simulink model "PID_MODEL"  (R2023b)
settings: Solver=FixedStepDiscrete  StartTime=0.0  StopTime=50  FixedStep=0.001  RelTol=1e-3
values from neighbouring files (symbols this model uses):
  ANG_A_D_CH1_1 = 0    [ini.m]
  ANG_A_D_CH1_2 = 0    [ini.m]
  ANG_A_D_CH1_3 = 0    [ini.m]
  ANG_A_D_CH1_4 = 0    [ini.m]
  ANG_A_D_CH1_5 = 0    [ini.m]
  ANG_A_D_CH1_6 = 0    [ini.m]
  ANG_A_D_CH1_7 = 0    [ini.m]
  ANG_A_D_CH2_1 = 0    [ini.m]
  ANG_A_D_CH2_2 = 0    [ini.m]
  ANG_A_D_CH2_3 = 0    [ini.m]
  ANG_A_D_CH2_4 = 0    [ini.m]
  ANG_A_D_CH2_5 = 0    [ini.m]
  ANG_A_D_CH2_6 = 0    [ini.m]
  ANG_A_D_CH2_7 = 0    [ini.m]
  ANG_A_I_CH1_1 = 0    [ini.m]
  ANG_A_I_CH1_2 = 0    [ini.m]
  ANG_A_I_CH1_3 = 0    [ini.m]
  ANG_A_I_CH1_4 = 0    [ini.m]
  ANG_A_I_CH1_5 = 0    [ini.m]
  ANG_A_I_CH1_6 = 0    [ini.m]
  ANG_A_I_CH1_7 = 0    [ini.m]
  ANG_A_I_CH2_1 = 0    [ini.m]
  ANG_A_I_CH2_2 = 0    [ini.m]
  ANG_A_I_CH2_3 = 0    [ini.m]
  ANG_A_I_CH2_4 = 0    [ini.m]
  ANG_A_I_CH2_5 = 0    [ini.m]
  ANG_A_I_CH2_6 = 0    [ini.m]
  ANG_A_I_CH2_7 = 0    [ini.m]
  ANG_A_P_CH1_1 = 0    [ini.m]
  ANG_A_P_CH1_2 = 0    [ini.m]
  ANG_A_P_CH1_3 = 0    [ini.m]
  ANG_A_P_CH1_4 = 0    [ini.m]
  ANG_A_P_CH1_5 = 0    [ini.m]
  ANG_A_P_CH1_6 = 0    [ini.m]
  ANG_A_P_CH1_7 = 0    [ini.m]
  ANG_A_P_CH2_1 = 0    [ini.m]
  ANG_A_P_CH2_2 = 0    [ini.m]
  ANG_A_P_CH2_3 = 0    [ini.m]
  ANG_A_P_CH2_4 = 0    [ini.m]
  ANG_A_P_CH2_5 = 0    [ini.m]
  ANG_A_P_CH2_6 = 0    [ini.m]
  ANG_A_P_CH2_7 = 0    [ini.m]
  ANG_S_D_CH1_1 = 0    [ini.m]
  ANG_S_D_CH1_2 = 0    [ini.m]
  ANG_S_D_CH1_3 = 0    [ini.m]
  ANG_S_D_CH1_4 = 0    [ini.m]
  ANG_S_D_CH1_5 = 0    [ini.m]
  ANG_S_D_CH1_6 = 0    [ini.m]
  ANG_S_D_CH1_7 = 0    [ini.m]
  ANG_S_D_CH2_1 = 0    [ini.m]
  ANG_S_D_CH2_2 = 0    [ini.m]
  ANG_S_D_CH2_3 = 0    [ini.m]
  ANG_S_D_CH2_4 = 0    [ini.m]
  ANG_S_D_CH2_5 = 0    [ini.m]
  ANG_S_D_CH2_6 = 0    [ini.m]
  ANG_S_D_CH2_7 = 0    [ini.m]
  ANG_S_I_CH1_1 = 0    [ini.m]
  ANG_S_I_CH1_2 = 0    [ini.m]
  ANG_S_I_CH1_3 = 0    [ini.m]
  ANG_S_I_CH1_4 = 0    [ini.m]
  ANG_S_I_CH1_5 = 0    [ini.m]
  ANG_S_I_CH1_6 = 0    [ini.m]
  ANG_S_I_CH1_7 = 0    [ini.m]
  ANG_S_I_CH2_1 = 0    [ini.m]
  ANG_S_I_CH2_2 = 0    [ini.m]
  ANG_S_I_CH2_3 = 0    [ini.m]
  ANG_S_I_CH2_4 = 0    [ini.m]
  ANG_S_I_CH2_5 = 0    [ini.m]
  ANG_S_I_CH2_6 = 0    [ini.m]
  ANG_S_I_CH2_7 = 0    [ini.m]
  ANG_S_P_CH1_1 = 0    [ini.m]
  ANG_S_P_CH1_2 = 0    [ini.m]
  ANG_S_P_CH1_3 = 0    [ini.m]
  ANG_S_P_CH1_4 = 0    [ini.m]
  ANG_S_P_CH1_5 = 0    [ini.m]
  ANG_S_P_CH1_6 = 0    [ini.m]
  ANG_S_P_CH1_7 = 0    [ini.m]
  ANG_S_P_CH2_1 = 0    [ini.m]
  ANG_S_P_CH2_2 = 0    [ini.m]
  ANG_S_P_CH2_3 = 0    [ini.m]
  ANG_S_P_CH2_4 = 0    [ini.m]
  ANG_S_P_CH2_5 = 0    [ini.m]
  ANG_S_P_CH2_6 = 0    [ini.m]
  ANG_S_P_CH2_7 = 0    [ini.m]
  DEADBAND_CH1_1 = 500    [ini.m]
  DEADBAND_CH1_2 = 500    [ini.m]
  DEADBAND_CH1_3 = 500    [ini.m]
  DEADBAND_CH1_4 = 500    [ini.m]
  DEADBAND_CH1_5 = 500    [ini.m]
  DEADBAND_CH1_6 = 500    [ini.m]
  DEADBAND_CH1_7 = 500    [ini.m]
  DEADBAND_CH2_1 = 500    [ini.m]
  DEADBAND_CH2_2 = 500    [ini.m]
  DEADBAND_CH2_3 = 500    [ini.m]
  DEADBAND_CH2_4 = 500    [ini.m]
  DEADBAND_CH2_5 = 500    [ini.m]
  DEADBAND_CH2_6 = 500    [ini.m]
  DEADBAND_CH2_7 = 500    [ini.m]
  SPD_D_CH1_1 = 0    [ini.m]
  SPD_D_CH1_2 = 0    [ini.m]
  SPD_D_CH1_3 = 0    [ini.m]
  SPD_D_CH1_4 = 0    [ini.m]
  SPD_D_CH1_5 = 0    [ini.m]
  SPD_D_CH1_6 = 0    [ini.m]
  SPD_D_CH1_7 = 0    [ini.m]
  SPD_D_CH2_1 = 0    [ini.m]
  SPD_D_CH2_2 = 0    [ini.m]
  SPD_D_CH2_3 = 0    [ini.m]
  SPD_D_CH2_4 = 0    [ini.m]
  SPD_D_CH2_5 = 0    [ini.m]
  SPD_D_CH2_6 = 0    [ini.m]
  SPD_D_CH2_7 = 0    [ini.m]
  SPD_I_CH1_1 = 0    [ini.m]
  SPD_I_CH1_2 = 0    [ini.m]
  SPD_I_CH1_3 = 0    [ini.m]
  SPD_I_CH1_4 = 0    [ini.m]
  SPD_I_CH1_5 = 0    [ini.m]
  SPD_I_CH1_6 = 0    [ini.m]
  SPD_I_CH1_7 = 0    [ini.m]
  SPD_I_CH2_1 = 0    [ini.m]
  ... (+34 more)
libraries: slpidlib x42
(part 5 of 5)

== system PID_MODEL/Yaw_CH2_5/If Action_speed Subsystem ==
  yaw_speed_rpm : Inport  OutDataTypeStr=single
  yaw_target : Inport  Port=2  OutDataTypeStr=single
  Action Port : ActionPort  ActionPortLabel=case [ 1 ]:
  Discrete PID Controller1 : slpidlib/PID Controller  Controller=PID  Form=Parallel  TimeDomain=Discrete-time  UseExternalTs=off  SampleTime=-1  IntegratorMethod=Forward Euler  FilterMethod=Forward Euler  ControllerParametersSource=internal  P=SPD_P_CH2_5  I=SPD_I_CH2_5  UseKiTs=off  D=SPD_D_CH2_5  N=100  UseFilter=on  TunerSelectOption=Transfer Function Based (PID Tuner App)  InitialConditionSource=internal  InitialConditionForIntegrator=0  InitialConditionForFilter=0  DifferentiatorICPrevScaledInput=0  ExternalReset=none  TrackingMode=off  Kt=1  LimitOutput=on  SatLimitsSource=internal  UpperSaturationLimit=16384  LowerSaturationLimit=-16384  LinearizeAsGain=off  AntiWindupMode=none  Kb=1  LimitIntegrator=off  UpperIntegratorSaturationLimit=inf  LowerIntegratorSaturationLimit=-inf  POutMin=[]  POutMax=[]  IOutMin=[]  IOutMax=[]  DOutMin=[]  DOutMax=[]  NOutMin=[]  NOutMax=[]  SumOutMin=[]  SumOutMax=[]  SaturationOutMin=[]  SaturationOutMax=[]  PParamMin=[]  PParamMax=[]  IParamMin=[]  IParamMax=[]  DParamMin=[]  DParamMax=[]  NParamMin=[]  NParamMax=[]  KbParamMin=[]  KbParamMax=[]  KtParamMin=[]  KtParamMax=[]  KbOutMin=[]  KbOutMax=[]  KtOutMin=[]  KtOutMax=[]  IntegratorOutMin=[]  IntegratorOutMax=[]  FilterOutMin=[]  FilterOutMax=[]  SumI1OutMin=[]  SumI1OutMax=[]  SumI2OutMin=[]  SumI2OutMax=[]  SumI3OutMin=[]  SumI3OutMax=[]  SumI4OutMin=[]  SumI4OutMax=[]  SumDOutMin=[]  SumDOutMax=[]  DifferentiatorOutMin=[]  DifferentiatorOutMax=[]  FilterDiffOutCoefMin=[]  FilterDiffOutCoefMax=[]  ReciprocalOutMin=[]  ReciprocalOutMax=[]  SumDenOutMin=[]  SumDenOutMax=[]  SumNumOutMin=[]  SumNumOutMax=[]  DivideOutMin=[]  DivideOutMax=[]  UdiffTsProdOutMin=[]  UdiffTsProdOutMax=[]  NTsProdOutMin=[]  NTsProdOutMax=[]  UintegralTsProdOutMin=[]  UintegralTsProdOutMax=[]  UngainTsProdOutMin=[]  UngainTsProdOutMax=[]  ClampingZeroOutDataTypeStr=Inherit: Inherit via back propagation  ClampingZeroOutMin=[]  ClampingZeroOutMax=[]  FilterDenConstantOutDataTypeStr=Inherit: Inherit via back propagation  FilterDenConstantOutMin=[]  FilterDenConstantOutMax=[]  PCopyOutDataTypeStr=Inherit: Inherit via back propagation  PCopyOutMin=[]  PCopyOutMax=[]  NCopyOutDataTypeStr=Inherit: Inherit via back propagation  NCopyOutMin=[]  NCopyOutMax=[]  IntegratorContinuousStateAttributes=''  IntegratorStateMustResolveToSignalObject=off  IntegratorRTWStateStorageClass=Auto  FilterContinuousStateAttributes=''  FilterStateMustResolveToSignalObject=off  FilterRTWStateStorageClass=Auto  ParallelPVariant=InternalParameters  IdealPVariant=Disabled  IVariant=InternalParameters  DVariant=InternalParameters  IntegratorVariant=Discrete  SatVariant=Enabled  AWVariant=Passthrough  PCopyVariant=Disabled  TRVariant=Disabled  FdbkBlocksVariant=Forward  IdealPFdbkVariant=Disabled  SatFdbkVariant=Disabled  DerivativeFilterVariant=ForwardEulerFilter  NVariant=InternalParameters  NCopyVariant=Disabled  FilterICVariant=InternalICsFilter  IntegratorICVariant=InternalICs  ExternalResetVariant=Disabled  TRSumVariant=Passthrough  SumFdbkVariant=Disabled  SumVariant=Sum_PID  TsampFilterVariant=InternalTs  TsampNgainVariant=Passthrough  TsampIntegralVariant=Disabled_SignalSpec  ExternalSaturationOutDataTypeStr=Inherit: Same as second input
      settings: LibrarySourceBlock=simulink/Discrete/Discrete PID Controller
  Sum : Sum  Inputs=|+-  OutDataTypeStr=single
  Out1 : Outport  OutDataTypeStr=single
  wires:
  yaw_speed_rpm/1 -> Sum/2
  yaw_target/1 -> Sum/1
  Sum/1 -> Discrete PID Controller1/1
  Discrete PID Controller1/1 -> Out1/1

== system PID_MODEL/Yaw_CH2_5/If Action_speed Subsystem1 ==
  yaw_speed_rpm : Inport  OutDataTypeStr=single
  yaw_target : Inport  Port=2  OutDataTypeStr=single
  yaw_ecd : Inport  Port=3  OutDataTypeStr=single
  yaw_last_ecd : Inport  Port=4  OutDataTypeStr=single
  yaw_circle : Inport  Port=5  OutDataTypeStr=single
  Action Port : ActionPort  ActionPortLabel=case [ 2 ]:
  Abs : Abs  OutDataTypeStr=single  SaturateOnIntegerOverflow=off
  Chart1 : Stateflow chart  TreatAsAtomicUnit=on
  Constant : Constant  Value=0  OutDataTypeStr=single
  Discrete PID Controller : slpidlib/PID Controller  Controller=PID  Form=Parallel  TimeDomain=Discrete-time  UseExternalTs=off  SampleTime=-1  IntegratorMethod=Forward Euler  FilterMethod=Forward Euler  ControllerParametersSource=internal  P=ANG_S_P_CH2_5  I=ANG_S_I_CH2_5  UseKiTs=off  D=ANG_S_D_CH2_5  N=100  UseFilter=on  TunerSelectOption=Transfer Function Based (PID Tuner App)  InitialConditionSource=internal  InitialConditionForIntegrator=0  InitialConditionForFilter=0  DifferentiatorICPrevScaledInput=0  ExternalReset=none  TrackingMode=off  Kt=1  LimitOutput=on  SatLimitsSource=internal  UpperSaturationLimit=16384  LowerSaturationLimit=-16384  LinearizeAsGain=off  AntiWindupMode=none  Kb=1  LimitIntegrator=off  UpperIntegratorSaturationLimit=2000  LowerIntegratorSaturationLimit=-2000  POutMin=[]  POutMax=[]  IOutMin=[]  IOutMax=[]  DOutMin=[]  DOutMax=[]  NOutMin=[]  NOutMax=[]  SumOutMin=[]  SumOutMax=[]  SaturationOutMin=[]  SaturationOutMax=[]  PParamMin=[]  PParamMax=[]  IParamMin=[]  IParamMax=[]  DParamMin=[]  DParamMax=[]  NParamMin=[]  NParamMax=[]  KbParamMin=[]  KbParamMax=[]  KtParamMin=[]  KtParamMax=[]  KbOutMin=[]  KbOutMax=[]  KtOutMin=[]  KtOutMax=[]  IntegratorOutMin=[]  IntegratorOutMax=[]  FilterOutMin=[]  FilterOutMax=[]  SumI1OutMin=[]  SumI1OutMax=[]  SumI2OutMin=[]  SumI2OutMax=[]  SumI3OutMin=[]  SumI3OutMax=[]  SumI4OutMin=[]  SumI4OutMax=[]  SumDOutMin=[]  SumDOutMax=[]  DifferentiatorOutMin=[]  DifferentiatorOutMax=[]  FilterDiffOutCoefMin=[]  FilterDiffOutCoefMax=[]  ReciprocalOutMin=[]  ReciprocalOutMax=[]  SumDenOutMin=[]  SumDenOutMax=[]  SumNumOutMin=[]  SumNumOutMax=[]  DivideOutMin=[]  DivideOutMax=[]  UdiffTsProdOutMin=[]  UdiffTsProdOutMax=[]  NTsProdOutMin=[]  NTsProdOutMax=[]  UintegralTsProdOutMin=[]  UintegralTsProdOutMax=[]  UngainTsProdOutMin=[]  UngainTsProdOutMax=[]  ClampingZeroOutDataTypeStr=Inherit: Inherit via back propagation  ClampingZeroOutMin=[]  ClampingZeroOutMax=[]  FilterDenConstantOutDataTypeStr=Inherit: Inherit via back propagation  FilterDenConstantOutMin=[]  FilterDenConstantOutMax=[]  PCopyOutDataTypeStr=Inherit: Inherit via back propagation  PCopyOutMin=[]  PCopyOutMax=[]  NCopyOutDataTypeStr=Inherit: Inherit via back propagation  NCopyOutMin=[]  NCopyOutMax=[]  IntegratorContinuousStateAttributes=''  IntegratorStateMustResolveToSignalObject=off  IntegratorRTWStateStorageClass=Auto  FilterContinuousStateAttributes=''  FilterStateMustResolveToSignalObject=off  FilterRTWStateStorageClass=Auto  ParallelPVariant=InternalParameters  IdealPVariant=Disabled  IVariant=InternalParameters  DVariant=InternalParameters  IntegratorVariant=Discrete  SatVariant=Enabled  AWVariant=Passthrough  PCopyVariant=Disabled  TRVariant=Disabled  FdbkBlocksVariant=Forward  IdealPFdbkVariant=Disabled  SatFdbkVariant=Disabled  DerivativeFilterVariant=ForwardEulerFilter  NVariant=InternalParameters  NCopyVariant=Disabled  FilterICVariant=InternalICsFilter  IntegratorICVariant=InternalICs  ExternalResetVariant=Disabled  TRSumVariant=Passthrough  SumFdbkVariant=Disabled  SumVariant=Sum_PID  TsampFilterVariant=InternalTs  TsampNgainVariant=Passthrough  TsampIntegralVariant=Disabled_SignalSpec  ExternalSaturationOutDataTypeStr=Inherit: Same as second input
      settings: LibrarySourceBlock=simulink/Discrete/Discrete PID Controller
  Discrete PID Controller1 : slpidlib/PID Controller  Controller=PID  Form=Parallel  TimeDomain=Discrete-time  UseExternalTs=off  SampleTime=-1  IntegratorMethod=Forward Euler  FilterMethod=Forward Euler  ControllerParametersSource=internal  P=ANG_A_P_CH2_5  I=ANG_A_I_CH2_5  UseKiTs=off  D=ANG_A_D_CH2_5  N=100  UseFilter=on  TunerSelectOption=Transfer Function Based (PID Tuner App)  InitialConditionSource=internal  InitialConditionForIntegrator=0  InitialConditionForFilter=0  DifferentiatorICPrevScaledInput=0  ExternalReset=none  TrackingMode=off  Kt=1  LimitOutput=on  SatLimitsSource=internal  UpperSaturationLimit=16384  LowerSaturationLimit=-16384  LinearizeAsGain=off  AntiWindupMode=none  Kb=1  LimitIntegrator=off  UpperIntegratorSaturationLimit=500  LowerIntegratorSaturationLimit=-500  POutMin=[]  POutMax=[]  IOutMin=[]  IOutMax=[]  DOutMin=[]  DOutMax=[]  NOutMin=[]  NOutMax=[]  SumOutMin=[]  SumOutMax=[]  SaturationOutMin=[]  SaturationOutMax=[]  PParamMin=[]  PParamMax=[]  IParamMin=[]  IParamMax=[]  DParamMin=[]  DParamMax=[]  NParamMin=[]  NParamMax=[]  KbParamMin=[]  KbParamMax=[]  KtParamMin=[]  KtParamMax=[]  KbOutMin=[]  KbOutMax=[]  KtOutMin=[]  KtOutMax=[]  IntegratorOutMin=[]  IntegratorOutMax=[]  FilterOutMin=[]  FilterOutMax=[]  SumI1OutMin=[]  SumI1OutMax=[]  SumI2OutMin=[]  SumI2OutMax=[]  SumI3OutMin=[]  SumI3OutMax=[]  SumI4OutMin=[]  SumI4OutMax=[]  SumDOutMin=[]  SumDOutMax=[]  DifferentiatorOutMin=[]  DifferentiatorOutMax=[]  FilterDiffOutCoefMin=[]  FilterDiffOutCoefMax=[]  ReciprocalOutMin=[]  ReciprocalOutMax=[]  SumDenOutMin=[]  SumDenOutMax=[]  SumNumOutMin=[]  SumNumOutMax=[]  DivideOutMin=[]  DivideOutMax=[]  UdiffTsProdOutMin=[]  UdiffTsProdOutMax=[]  NTsProdOutMin=[]  NTsProdOutMax=[]  UintegralTsProdOutMin=[]  UintegralTsProdOutMax=[]  UngainTsProdOutMin=[]  UngainTsProdOutMax=[]  ClampingZeroOutDataTypeStr=Inherit: Inherit via back propagation  ClampingZeroOutMin=[]  ClampingZeroOutMax=[]  FilterDenConstantOutDataTypeStr=Inherit: Inherit via back propagation  FilterDenConstantOutMin=[]  FilterDenConstantOutMax=[]  PCopyOutDataTypeStr=Inherit: Inherit via back propagation  PCopyOutMin=[]  PCopyOutMax=[]  NCopyOutDataTypeStr=Inherit: Inherit via back propagation  NCopyOutMin=[]  NCopyOutMax=[]  IntegratorContinuousStateAttributes=''  IntegratorStateMustResolveToSignalObject=off  IntegratorRTWStateStorageClass=Auto  FilterContinuousStateAttributes=''  FilterStateMustResolveToSignalObject=off  FilterRTWStateStorageClass=Auto  ParallelPVariant=InternalParameters  IdealPVariant=Disabled  IVariant=InternalParameters  DVariant=InternalParameters  IntegratorVariant=Discrete  SatVariant=Enabled  AWVariant=Passthrough  PCopyVariant=Disabled  TRVariant=Disabled  FdbkBlocksVariant=Forward  IdealPFdbkVariant=Disabled  SatFdbkVariant=Disabled  DerivativeFilterVariant=ForwardEulerFilter  NVariant=InternalParameters  NCopyVariant=Disabled  FilterICVariant=InternalICsFilter  IntegratorICVariant=InternalICs  ExternalResetVariant=Disabled  TRSumVariant=Passthrough  SumFdbkVariant=Disabled  SumVariant=Sum_PID  TsampFilterVariant=InternalTs  TsampNgainVariant=Passthrough  TsampIntegralVariant=Disabled_SignalSpec  ExternalSaturationOutDataTypeStr=Inherit: Same as second input
      settings: LibrarySourceBlock=simulink/Discrete/Discrete PID Controller
  Gain : Gain  Gain=8191  OutDataTypeStr=single
  Multiply : Gain  Gain=TRANS_CH2_5  OutDataTypeStr=single
  Sum : Sum  Inputs=|+-  OutDataTypeStr=single
  Sum1 : Sum  Inputs=|+-  OutDataTypeStr=single
  Sum2 : Sum  Inputs=|++  OutDataTypeStr=single
  Sum3 : Sum  Inputs=|+-  OutDataTypeStr=single
  Sum4 : Sum  Inputs=|++  OutDataTypeStr=single
  Switch1 : Switch  Criteria=u2 > Threshold  Threshold=DEADBAND_CH2_5  OutDataTypeStr=single  SaturateOnIntegerOverflow=off  InputSameDT=off
  Switch2 : Switch  Criteria=u2 > Threshold  Threshold=DEADBAND_CH2_5  OutDataTypeStr=single  SaturateOnIntegerOverflow=off  InputSameDT=off
  Out1 : Outport  OutDataTypeStr=single
  yaw_circle_out : Outport  Port=2  OutDataTypeStr=single
  wires:
  yaw_target/1 -> Sum/1
  Discrete PID Controller1/1 -> Multiply/1
  yaw_circle/1 -> Sum4/2, Gain/1
  Gain/1 -> Sum2/1
  yaw_ecd/1 -> Sum2/2, Sum3/1
  Sum2/1 -> Sum/2
  yaw_last_ecd/1 -> Sum3/2
  Sum3/1 -> Chart1/1(u1)
  Chart1/1(u2) -> Sum4/1
  Sum4/1 -> yaw_circle_out/1
  Multiply/1 -> Sum1/1
  Sum1/1 -> Switch1/1
  yaw_speed_rpm/1 -> Sum1/2
  Discrete PID Controller/1 -> Out1/1
  Switch1/1 -> Discrete PID Controller/1
  Abs/1 -> Switch2/2, Switch1/2
  Constant/1 -> Switch2/3, Switch1/3
  Sum/1 -> Switch2/1, Abs/1
  Switch2/1 -> Discrete PID Controller1/1

== system PID_MODEL/Yaw_CH2_6/If Action_speed Subsystem ==
  yaw_speed_rpm : Inport  OutDataTypeStr=single
  yaw_target : Inport  Port=2  OutDataTypeStr=single
  Action Port : ActionPort  ActionPortLabel=case [ 1 ]:
  Discrete PID Controller1 : slpidlib/PID Controller  Controller=PID  Form=Parallel  TimeDomain=Discrete-time  UseExternalTs=off  SampleTime=-1  IntegratorMethod=Forward Euler  FilterMethod=Forward Euler  ControllerParametersSource=internal  P=SPD_P_CH2_6  I=SPD_I_CH2_6  UseKiTs=off  D=SPD_D_CH2_6  N=100  UseFilter=on  TunerSelectOption=Transfer Function Based (PID Tuner App)  InitialConditionSource=internal  InitialConditionForIntegrator=0  InitialConditionForFilter=0  DifferentiatorICPrevScaledInput=0  ExternalReset=none  TrackingMode=off  Kt=1  LimitOutput=on  SatLimitsSource=internal  UpperSaturationLimit=16384  LowerSaturationLimit=-16384  LinearizeAsGain=off  AntiWindupMode=none  Kb=1  LimitIntegrator=off  UpperIntegratorSaturationLimit=inf  LowerIntegratorSaturationLimit=-inf  POutMin=[]  POutMax=[]  IOutMin=[]  IOutMax=[]  DOutMin=[]  DOutMax=[]  NOutMin=[]  NOutMax=[]  SumOutMin=[]  SumOutMax=[]  SaturationOutMin=[]  SaturationOutMax=[]  PParamMin=[]  PParamMax=[]  IParamMin=[]  IParamMax=[]  DParamMin=[]  DParamMax=[]  NParamMin=[]  NParamMax=[]  KbParamMin=[]  KbParamMax=[]  KtParamMin=[]  KtParamMax=[]  KbOutMin=[]  KbOutMax=[]  KtOutMin=[]  KtOutMax=[]  IntegratorOutMin=[]  IntegratorOutMax=[]  FilterOutMin=[]  FilterOutMax=[]  SumI1OutMin=[]  SumI1OutMax=[]  SumI2OutMin=[]  SumI2OutMax=[]  SumI3OutMin=[]  SumI3OutMax=[]  SumI4OutMin=[]  SumI4OutMax=[]  SumDOutMin=[]  SumDOutMax=[]  DifferentiatorOutMin=[]  DifferentiatorOutMax=[]  FilterDiffOutCoefMin=[]  FilterDiffOutCoefMax=[]  ReciprocalOutMin=[]  ReciprocalOutMax=[]  SumDenOutMin=[]  SumDenOutMax=[]  SumNumOutMin=[]  SumNumOutMax=[]  DivideOutMin=[]  DivideOutMax=[]  UdiffTsProdOutMin=[]  UdiffTsProdOutMax=[]  NTsProdOutMin=[]  NTsProdOutMax=[]  UintegralTsProdOutMin=[]  UintegralTsProdOutMax=[]  UngainTsProdOutMin=[]  UngainTsProdOutMax=[]  ClampingZeroOutDataTypeStr=Inherit: Inherit via back propagation  ClampingZeroOutMin=[]  ClampingZeroOutMax=[]  FilterDenConstantOutDataTypeStr=Inherit: Inherit via back propagation  FilterDenConstantOutMin=[]  FilterDenConstantOutMax=[]  PCopyOutDataTypeStr=Inherit: Inherit via back propagation  PCopyOutMin=[]  PCopyOutMax=[]  NCopyOutDataTypeStr=Inherit: Inherit via back propagation  NCopyOutMin=[]  NCopyOutMax=[]  IntegratorContinuousStateAttributes=''  IntegratorStateMustResolveToSignalObject=off  IntegratorRTWStateStorageClass=Auto  FilterContinuousStateAttributes=''  FilterStateMustResolveToSignalObject=off  FilterRTWStateStorageClass=Auto  ParallelPVariant=InternalParameters  IdealPVariant=Disabled  IVariant=InternalParameters  DVariant=InternalParameters  IntegratorVariant=Discrete  SatVariant=Enabled  AWVariant=Passthrough  PCopyVariant=Disabled  TRVariant=Disabled  FdbkBlocksVariant=Forward  IdealPFdbkVariant=Disabled  SatFdbkVariant=Disabled  DerivativeFilterVariant=ForwardEulerFilter  NVariant=InternalParameters  NCopyVariant=Disabled  FilterICVariant=InternalICsFilter  IntegratorICVariant=InternalICs  ExternalResetVariant=Disabled  TRSumVariant=Passthrough  SumFdbkVariant=Disabled  SumVariant=Sum_PID  TsampFilterVariant=InternalTs  TsampNgainVariant=Passthrough  TsampIntegralVariant=Disabled_SignalSpec  ExternalSaturationOutDataTypeStr=Inherit: Same as second input
      settings: LibrarySourceBlock=simulink/Discrete/Discrete PID Controller
  Sum : Sum  Inputs=|+-  OutDataTypeStr=single
  Out1 : Outport  OutDataTypeStr=single
  wires:
  yaw_speed_rpm/1 -> Sum/2
  yaw_target/1 -> Sum/1
  Sum/1 -> Discrete PID Controller1/1
  Discrete PID Controller1/1 -> Out1/1

== system PID_MODEL/Yaw_CH2_6/If Action_speed Subsystem1 ==
  yaw_speed_rpm : Inport  OutDataTypeStr=single
  yaw_target : Inport  Port=2  OutDataTypeStr=single
  yaw_ecd : Inport  Port=3  OutDataTypeStr=single
  yaw_last_ecd : Inport  Port=4  OutDataTypeStr=single
  yaw_circle : Inport  Port=5  OutDataTypeStr=single
  Action Port : ActionPort  ActionPortLabel=case [ 2 ]:
  Abs : Abs  OutDataTypeStr=single  SaturateOnIntegerOverflow=off
  Chart1 : Stateflow chart  TreatAsAtomicUnit=on
  Constant : Constant  Value=0  OutDataTypeStr=single
  Discrete PID Controller : slpidlib/PID Controller  Controller=PID  Form=Parallel  TimeDomain=Discrete-time  UseExternalTs=off  SampleTime=-1  IntegratorMethod=Forward Euler  FilterMethod=Forward Euler  ControllerParametersSource=internal  P=ANG_S_P_CH2_6  I=ANG_S_I_CH2_6  UseKiTs=off  D=ANG_S_D_CH2_6  N=100  UseFilter=on  TunerSelectOption=Transfer Function Based (PID Tuner App)  InitialConditionSource=internal  InitialConditionForIntegrator=0  InitialConditionForFilter=0  DifferentiatorICPrevScaledInput=0  ExternalReset=none  TrackingMode=off  Kt=1  LimitOutput=on  SatLimitsSource=internal  UpperSaturationLimit=16384  LowerSaturationLimit=-16384  LinearizeAsGain=off  AntiWindupMode=none  Kb=1  LimitIntegrator=off  UpperIntegratorSaturationLimit=2000  LowerIntegratorSaturationLimit=-2000  POutMin=[]  POutMax=[]  IOutMin=[]  IOutMax=[]  DOutMin=[]  DOutMax=[]  NOutMin=[]  NOutMax=[]  SumOutMin=[]  SumOutMax=[]  SaturationOutMin=[]  SaturationOutMax=[]  PParamMin=[]  PParamMax=[]  IParamMin=[]  IParamMax=[]  DParamMin=[]  DParamMax=[]  NParamMin=[]  NParamMax=[]  KbParamMin=[]  KbParamMax=[]  KtParamMin=[]  KtParamMax=[]  KbOutMin=[]  KbOutMax=[]  KtOutMin=[]  KtOutMax=[]  IntegratorOutMin=[]  IntegratorOutMax=[]  FilterOutMin=[]  FilterOutMax=[]  SumI1OutMin=[]  SumI1OutMax=[]  SumI2OutMin=[]  SumI2OutMax=[]  SumI3OutMin=[]  SumI3OutMax=[]  SumI4OutMin=[]  SumI4OutMax=[]  SumDOutMin=[]  SumDOutMax=[]  DifferentiatorOutMin=[]  DifferentiatorOutMax=[]  FilterDiffOutCoefMin=[]  FilterDiffOutCoefMax=[]  ReciprocalOutMin=[]  ReciprocalOutMax=[]  SumDenOutMin=[]  SumDenOutMax=[]  SumNumOutMin=[]  SumNumOutMax=[]  DivideOutMin=[]  DivideOutMax=[]  UdiffTsProdOutMin=[]  UdiffTsProdOutMax=[]  NTsProdOutMin=[]  NTsProdOutMax=[]  UintegralTsProdOutMin=[]  UintegralTsProdOutMax=[]  UngainTsProdOutMin=[]  UngainTsProdOutMax=[]  ClampingZeroOutDataTypeStr=Inherit: Inherit via back propagation  ClampingZeroOutMin=[]  ClampingZeroOutMax=[]  FilterDenConstantOutDataTypeStr=Inherit: Inherit via back propagation  FilterDenConstantOutMin=[]  FilterDenConstantOutMax=[]  PCopyOutDataTypeStr=Inherit: Inherit via back propagation  PCopyOutMin=[]  PCopyOutMax=[]  NCopyOutDataTypeStr=Inherit: Inherit via back propagation  NCopyOutMin=[]  NCopyOutMax=[]  IntegratorContinuousStateAttributes=''  IntegratorStateMustResolveToSignalObject=off  IntegratorRTWStateStorageClass=Auto  FilterContinuousStateAttributes=''  FilterStateMustResolveToSignalObject=off  FilterRTWStateStorageClass=Auto  ParallelPVariant=InternalParameters  IdealPVariant=Disabled  IVariant=InternalParameters  DVariant=InternalParameters  IntegratorVariant=Discrete  SatVariant=Enabled  AWVariant=Passthrough  PCopyVariant=Disabled  TRVariant=Disabled  FdbkBlocksVariant=Forward  IdealPFdbkVariant=Disabled  SatFdbkVariant=Disabled  DerivativeFilterVariant=ForwardEulerFilter  NVariant=InternalParameters  NCopyVariant=Disabled  FilterICVariant=InternalICsFilter  IntegratorICVariant=InternalICs  ExternalResetVariant=Disabled  TRSumVariant=Passthrough  SumFdbkVariant=Disabled  SumVariant=Sum_PID  TsampFilterVariant=InternalTs  TsampNgainVariant=Passthrough  TsampIntegralVariant=Disabled_SignalSpec  ExternalSaturationOutDataTypeStr=Inherit: Same as second input
      settings: LibrarySourceBlock=simulink/Discrete/Discrete PID Controller
  Discrete PID Controller1 : slpidlib/PID Controller  Controller=PID  Form=Parallel  TimeDomain=Discrete-time  UseExternalTs=off  SampleTime=-1  IntegratorMethod=Forward Euler  FilterMethod=Forward Euler  ControllerParametersSource=internal  P=ANG_A_P_CH2_6  I=ANG_A_I_CH2_6  UseKiTs=off  D=ANG_A_D_CH2_6  N=100  UseFilter=on  TunerSelectOption=Transfer Function Based (PID Tuner App)  InitialConditionSource=internal  InitialConditionForIntegrator=0  InitialConditionForFilter=0  DifferentiatorICPrevScaledInput=0  ExternalReset=none  TrackingMode=off  Kt=1  LimitOutput=on  SatLimitsSource=internal  UpperSaturationLimit=16384  LowerSaturationLimit=-16384  LinearizeAsGain=off  AntiWindupMode=none  Kb=1  LimitIntegrator=off  UpperIntegratorSaturationLimit=500  LowerIntegratorSaturationLimit=-500  POutMin=[]  POutMax=[]  IOutMin=[]  IOutMax=[]  DOutMin=[]  DOutMax=[]  NOutMin=[]  NOutMax=[]  SumOutMin=[]  SumOutMax=[]  SaturationOutMin=[]  SaturationOutMax=[]  PParamMin=[]  PParamMax=[]  IParamMin=[]  IParamMax=[]  DParamMin=[]  DParamMax=[]  NParamMin=[]  NParamMax=[]  KbParamMin=[]  KbParamMax=[]  KtParamMin=[]  KtParamMax=[]  KbOutMin=[]  KbOutMax=[]  KtOutMin=[]  KtOutMax=[]  IntegratorOutMin=[]  IntegratorOutMax=[]  FilterOutMin=[]  FilterOutMax=[]  SumI1OutMin=[]  SumI1OutMax=[]  SumI2OutMin=[]  SumI2OutMax=[]  SumI3OutMin=[]  SumI3OutMax=[]  SumI4OutMin=[]  SumI4OutMax=[]  SumDOutMin=[]  SumDOutMax=[]  DifferentiatorOutMin=[]  DifferentiatorOutMax=[]  FilterDiffOutCoefMin=[]  FilterDiffOutCoefMax=[]  ReciprocalOutMin=[]  ReciprocalOutMax=[]  SumDenOutMin=[]  SumDenOutMax=[]  SumNumOutMin=[]  SumNumOutMax=[]  DivideOutMin=[]  DivideOutMax=[]  UdiffTsProdOutMin=[]  UdiffTsProdOutMax=[]  NTsProdOutMin=[]  NTsProdOutMax=[]  UintegralTsProdOutMin=[]  UintegralTsProdOutMax=[]  UngainTsProdOutMin=[]  UngainTsProdOutMax=[]  ClampingZeroOutDataTypeStr=Inherit: Inherit via back propagation  ClampingZeroOutMin=[]  ClampingZeroOutMax=[]  FilterDenConstantOutDataTypeStr=Inherit: Inherit via back propagation  FilterDenConstantOutMin=[]  FilterDenConstantOutMax=[]  PCopyOutDataTypeStr=Inherit: Inherit via back propagation  PCopyOutMin=[]  PCopyOutMax=[]  NCopyOutDataTypeStr=Inherit: Inherit via back propagation  NCopyOutMin=[]  NCopyOutMax=[]  IntegratorContinuousStateAttributes=''  IntegratorStateMustResolveToSignalObject=off  IntegratorRTWStateStorageClass=Auto  FilterContinuousStateAttributes=''  FilterStateMustResolveToSignalObject=off  FilterRTWStateStorageClass=Auto  ParallelPVariant=InternalParameters  IdealPVariant=Disabled  IVariant=InternalParameters  DVariant=InternalParameters  IntegratorVariant=Discrete  SatVariant=Enabled  AWVariant=Passthrough  PCopyVariant=Disabled  TRVariant=Disabled  FdbkBlocksVariant=Forward  IdealPFdbkVariant=Disabled  SatFdbkVariant=Disabled  DerivativeFilterVariant=ForwardEulerFilter  NVariant=InternalParameters  NCopyVariant=Disabled  FilterICVariant=InternalICsFilter  IntegratorICVariant=InternalICs  ExternalResetVariant=Disabled  TRSumVariant=Passthrough  SumFdbkVariant=Disabled  SumVariant=Sum_PID  TsampFilterVariant=InternalTs  TsampNgainVariant=Passthrough  TsampIntegralVariant=Disabled_SignalSpec  ExternalSaturationOutDataTypeStr=Inherit: Same as second input
      settings: LibrarySourceBlock=simulink/Discrete/Discrete PID Controller
  Gain : Gain  Gain=8191  OutDataTypeStr=single
  Multiply : Gain  Gain=TRANS_CH2_6  OutDataTypeStr=single
  Sum : Sum  Inputs=|+-  OutDataTypeStr=single
  Sum1 : Sum  Inputs=|+-  OutDataTypeStr=single
  Sum2 : Sum  Inputs=|++  OutDataTypeStr=single
  Sum3 : Sum  Inputs=|+-  OutDataTypeStr=single
  Sum4 : Sum  Inputs=|++  OutDataTypeStr=single
  Switch1 : Switch  Criteria=u2 > Threshold  Threshold=DEADBAND_CH2_6  OutDataTypeStr=single  SaturateOnIntegerOverflow=off  InputSameDT=off
  Switch2 : Switch  Criteria=u2 > Threshold  Threshold=DEADBAND_CH2_6  OutDataTypeStr=single  SaturateOnIntegerOverflow=off  InputSameDT=off
  Out1 : Outport  OutDataTypeStr=single
  yaw_circle_out : Outport  Port=2  OutDataTypeStr=single
  wires:
  yaw_target/1 -> Sum/1
  Discrete PID Controller1/1 -> Multiply/1
  yaw_circle/1 -> Sum4/2, Gain/1
  Gain/1 -> Sum2/1
  yaw_ecd/1 -> Sum2/2, Sum3/1
  Sum2/1 -> Sum/2
  yaw_last_ecd/1 -> Sum3/2
  Sum3/1 -> Chart1/1(u1)
  Chart1/1(u2) -> Sum4/1
  Sum4/1 -> yaw_circle_out/1
  Multiply/1 -> Sum1/1
  Sum1/1 -> Switch1/1
  yaw_speed_rpm/1 -> Sum1/2
  Discrete PID Controller/1 -> Out1/1
  Switch1/1 -> Discrete PID Controller/1
  Abs/1 -> Switch2/2, Switch1/2
  Constant/1 -> Switch2/3, Switch1/3
  Sum/1 -> Switch2/1, Abs/1
  Switch2/1 -> Discrete PID Controller1/1

== system PID_MODEL/Yaw_CH2_7/If Action_speed Subsystem ==
  yaw_speed_rpm : Inport  OutDataTypeStr=single
  yaw_target : Inport  Port=2  OutDataTypeStr=single
  Action Port : ActionPort  ActionPortLabel=case [ 1 ]:
  Discrete PID Controller1 : slpidlib/PID Controller  Controller=PID  Form=Parallel  TimeDomain=Discrete-time  UseExternalTs=off  SampleTime=-1  IntegratorMethod=Forward Euler  FilterMethod=Forward Euler  ControllerParametersSource=internal  P=SPD_P_CH2_7  I=SPD_I_CH2_7  UseKiTs=off  D=SPD_D_CH2_7  N=100  UseFilter=on  TunerSelectOption=Transfer Function Based (PID Tuner App)  InitialConditionSource=internal  InitialConditionForIntegrator=0  InitialConditionForFilter=0  DifferentiatorICPrevScaledInput=0  ExternalReset=none  TrackingMode=off  Kt=1  LimitOutput=on  SatLimitsSource=internal  UpperSaturationLimit=16384  LowerSaturationLimit=-16384  LinearizeAsGain=off  AntiWindupMode=none  Kb=1  LimitIntegrator=off  UpperIntegratorSaturationLimit=inf  LowerIntegratorSaturationLimit=-inf  POutMin=[]  POutMax=[]  IOutMin=[]  IOutMax=[]  DOutMin=[]  DOutMax=[]  NOutMin=[]  NOutMax=[]  SumOutMin=[]  SumOutMax=[]  SaturationOutMin=[]  SaturationOutMax=[]  PParamMin=[]  PParamMax=[]  IParamMin=[]  IParamMax=[]  DParamMin=[]  DParamMax=[]  NParamMin=[]  NParamMax=[]  KbParamMin=[]  KbParamMax=[]  KtParamMin=[]  KtParamMax=[]  KbOutMin=[]  KbOutMax=[]  KtOutMin=[]  KtOutMax=[]  IntegratorOutMin=[]  IntegratorOutMax=[]  FilterOutMin=[]  FilterOutMax=[]  SumI1OutMin=[]  SumI1OutMax=[]  SumI2OutMin=[]  SumI2OutMax=[]  SumI3OutMin=[]  SumI3OutMax=[]  SumI4OutMin=[]  SumI4OutMax=[]  SumDOutMin=[]  SumDOutMax=[]  DifferentiatorOutMin=[]  DifferentiatorOutMax=[]  FilterDiffOutCoefMin=[]  FilterDiffOutCoefMax=[]  ReciprocalOutMin=[]  ReciprocalOutMax=[]  SumDenOutMin=[]  SumDenOutMax=[]  SumNumOutMin=[]  SumNumOutMax=[]  DivideOutMin=[]  DivideOutMax=[]  UdiffTsProdOutMin=[]  UdiffTsProdOutMax=[]  NTsProdOutMin=[]  NTsProdOutMax=[]  UintegralTsProdOutMin=[]  UintegralTsProdOutMax=[]  UngainTsProdOutMin=[]  UngainTsProdOutMax=[]  ClampingZeroOutDataTypeStr=Inherit: Inherit via back propagation  ClampingZeroOutMin=[]  ClampingZeroOutMax=[]  FilterDenConstantOutDataTypeStr=Inherit: Inherit via back propagation  FilterDenConstantOutMin=[]  FilterDenConstantOutMax=[]  PCopyOutDataTypeStr=Inherit: Inherit via back propagation  PCopyOutMin=[]  PCopyOutMax=[]  NCopyOutDataTypeStr=Inherit: Inherit via back propagation  NCopyOutMin=[]  NCopyOutMax=[]  IntegratorContinuousStateAttributes=''  IntegratorStateMustResolveToSignalObject=off  IntegratorRTWStateStorageClass=Auto  FilterContinuousStateAttributes=''  FilterStateMustResolveToSignalObject=off  FilterRTWStateStorageClass=Auto  ParallelPVariant=InternalParameters  IdealPVariant=Disabled  IVariant=InternalParameters  DVariant=InternalParameters  IntegratorVariant=Discrete  SatVariant=Enabled  AWVariant=Passthrough  PCopyVariant=Disabled  TRVariant=Disabled  FdbkBlocksVariant=Forward  IdealPFdbkVariant=Disabled  SatFdbkVariant=Disabled  DerivativeFilterVariant=ForwardEulerFilter  NVariant=InternalParameters  NCopyVariant=Disabled  FilterICVariant=InternalICsFilter  IntegratorICVariant=InternalICs  ExternalResetVariant=Disabled  TRSumVariant=Passthrough  SumFdbkVariant=Disabled  SumVariant=Sum_PID  TsampFilterVariant=InternalTs  TsampNgainVariant=Passthrough  TsampIntegralVariant=Disabled_SignalSpec  ExternalSaturationOutDataTypeStr=Inherit: Same as second input
      settings: LibrarySourceBlock=simulink/Discrete/Discrete PID Controller
  Sum : Sum  Inputs=|+-  OutDataTypeStr=single
  Out1 : Outport  OutDataTypeStr=single
  wires:
  yaw_speed_rpm/1 -> Sum/2
  yaw_target/1 -> Sum/1
  Sum/1 -> Discrete PID Controller1/1
  Discrete PID Controller1/1 -> Out1/1

== system PID_MODEL/Yaw_CH2_7/If Action_speed Subsystem1 ==
  yaw_speed_rpm : Inport  OutDataTypeStr=single
  yaw_target : Inport  Port=2  OutDataTypeStr=single
  yaw_ecd : Inport  Port=3  OutDataTypeStr=single
  yaw_last_ecd : Inport  Port=4  OutDataTypeStr=single
  yaw_circle : Inport  Port=5  OutDataTypeStr=single
  Action Port : ActionPort  ActionPortLabel=case [ 2 ]:
  Abs : Abs  OutDataTypeStr=single  SaturateOnIntegerOverflow=off
  Chart1 : Stateflow chart  TreatAsAtomicUnit=on
  Constant : Constant  Value=0  OutDataTypeStr=single
  Discrete PID Controller : slpidlib/PID Controller  Controller=PID  Form=Parallel  TimeDomain=Discrete-time  UseExternalTs=off  SampleTime=-1  IntegratorMethod=Forward Euler  FilterMethod=Forward Euler  ControllerParametersSource=internal  P=ANG_S_P_CH2_7  I=ANG_S_I_CH2_7  UseKiTs=off  D=ANG_S_D_CH2_7  N=100  UseFilter=on  TunerSelectOption=Transfer Function Based (PID Tuner App)  InitialConditionSource=internal  InitialConditionForIntegrator=0  InitialConditionForFilter=0  DifferentiatorICPrevScaledInput=0  ExternalReset=none  TrackingMode=off  Kt=1  LimitOutput=on  SatLimitsSource=internal  UpperSaturationLimit=16384  LowerSaturationLimit=-16384  LinearizeAsGain=off  AntiWindupMode=none  Kb=1  LimitIntegrator=off  UpperIntegratorSaturationLimit=2000  LowerIntegratorSaturationLimit=-2000  POutMin=[]  POutMax=[]  IOutMin=[]  IOutMax=[]  DOutMin=[]  DOutMax=[]  NOutMin=[]  NOutMax=[]  SumOutMin=[]  SumOutMax=[]  SaturationOutMin=[]  SaturationOutMax=[]  PParamMin=[]  PParamMax=[]  IParamMin=[]  IParamMax=[]  DParamMin=[]  DParamMax=[]  NParamMin=[]  NParamMax=[]  KbParamMin=[]  KbParamMax=[]  KtParamMin=[]  KtParamMax=[]  KbOutMin=[]  KbOutMax=[]  KtOutMin=[]  KtOutMax=[]  IntegratorOutMin=[]  IntegratorOutMax=[]  FilterOutMin=[]  FilterOutMax=[]  SumI1OutMin=[]  SumI1OutMax=[]  SumI2OutMin=[]  SumI2OutMax=[]  SumI3OutMin=[]  SumI3OutMax=[]  SumI4OutMin=[]  SumI4OutMax=[]  SumDOutMin=[]  SumDOutMax=[]  DifferentiatorOutMin=[]  DifferentiatorOutMax=[]  FilterDiffOutCoefMin=[]  FilterDiffOutCoefMax=[]  ReciprocalOutMin=[]  ReciprocalOutMax=[]  SumDenOutMin=[]  SumDenOutMax=[]  SumNumOutMin=[]  SumNumOutMax=[]  DivideOutMin=[]  DivideOutMax=[]  UdiffTsProdOutMin=[]  UdiffTsProdOutMax=[]  NTsProdOutMin=[]  NTsProdOutMax=[]  UintegralTsProdOutMin=[]  UintegralTsProdOutMax=[]  UngainTsProdOutMin=[]  UngainTsProdOutMax=[]  ClampingZeroOutDataTypeStr=Inherit: Inherit via back propagation  ClampingZeroOutMin=[]  ClampingZeroOutMax=[]  FilterDenConstantOutDataTypeStr=Inherit: Inherit via back propagation  FilterDenConstantOutMin=[]  FilterDenConstantOutMax=[]  PCopyOutDataTypeStr=Inherit: Inherit via back propagation  PCopyOutMin=[]  PCopyOutMax=[]  NCopyOutDataTypeStr=Inherit: Inherit via back propagation  NCopyOutMin=[]  NCopyOutMax=[]  IntegratorContinuousStateAttributes=''  IntegratorStateMustResolveToSignalObject=off  IntegratorRTWStateStorageClass=Auto  FilterContinuousStateAttributes=''  FilterStateMustResolveToSignalObject=off  FilterRTWStateStorageClass=Auto  ParallelPVariant=InternalParameters  IdealPVariant=Disabled  IVariant=InternalParameters  DVariant=InternalParameters  IntegratorVariant=Discrete  SatVariant=Enabled  AWVariant=Passthrough  PCopyVariant=Disabled  TRVariant=Disabled  FdbkBlocksVariant=Forward  IdealPFdbkVariant=Disabled  SatFdbkVariant=Disabled  DerivativeFilterVariant=ForwardEulerFilter  NVariant=InternalParameters  NCopyVariant=Disabled  FilterICVariant=InternalICsFilter  IntegratorICVariant=InternalICs  ExternalResetVariant=Disabled  TRSumVariant=Passthrough  SumFdbkVariant=Disabled  SumVariant=Sum_PID  TsampFilterVariant=InternalTs  TsampNgainVariant=Passthrough  TsampIntegralVariant=Disabled_SignalSpec  ExternalSaturationOutDataTypeStr=Inherit: Same as second input
      settings: LibrarySourceBlock=simulink/Discrete/Discrete PID Controller
  Discrete PID Controller1 : slpidlib/PID Controller  Controller=PID  Form=Parallel  TimeDomain=Discrete-time  UseExternalTs=off  SampleTime=-1  IntegratorMethod=Forward Euler  FilterMethod=Forward Euler  ControllerParametersSource=internal  P=ANG_A_P_CH2_7  I=ANG_A_I_CH2_7  UseKiTs=off  D=ANG_A_D_CH2_7  N=100  UseFilter=on  TunerSelectOption=Transfer Function Based (PID Tuner App)  InitialConditionSource=internal  InitialConditionForIntegrator=0  InitialConditionForFilter=0  DifferentiatorICPrevScaledInput=0  ExternalReset=none  TrackingMode=off  Kt=1  LimitOutput=on  SatLimitsSource=internal  UpperSaturationLimit=16384  LowerSaturationLimit=-16384  LinearizeAsGain=off  AntiWindupMode=none  Kb=1  LimitIntegrator=off  UpperIntegratorSaturationLimit=500  LowerIntegratorSaturationLimit=-500  POutMin=[]  POutMax=[]  IOutMin=[]  IOutMax=[]  DOutMin=[]  DOutMax=[]  NOutMin=[]  NOutMax=[]  SumOutMin=[]  SumOutMax=[]  SaturationOutMin=[]  SaturationOutMax=[]  PParamMin=[]  PParamMax=[]  IParamMin=[]  IParamMax=[]  DParamMin=[]  DParamMax=[]  NParamMin=[]  NParamMax=[]  KbParamMin=[]  KbParamMax=[]  KtParamMin=[]  KtParamMax=[]  KbOutMin=[]  KbOutMax=[]  KtOutMin=[]  KtOutMax=[]  IntegratorOutMin=[]  IntegratorOutMax=[]  FilterOutMin=[]  FilterOutMax=[]  SumI1OutMin=[]  SumI1OutMax=[]  SumI2OutMin=[]  SumI2OutMax=[]  SumI3OutMin=[]  SumI3OutMax=[]  SumI4OutMin=[]  SumI4OutMax=[]  SumDOutMin=[]  SumDOutMax=[]  DifferentiatorOutMin=[]  DifferentiatorOutMax=[]  FilterDiffOutCoefMin=[]  FilterDiffOutCoefMax=[]  ReciprocalOutMin=[]  ReciprocalOutMax=[]  SumDenOutMin=[]  SumDenOutMax=[]  SumNumOutMin=[]  SumNumOutMax=[]  DivideOutMin=[]  DivideOutMax=[]  UdiffTsProdOutMin=[]  UdiffTsProdOutMax=[]  NTsProdOutMin=[]  NTsProdOutMax=[]  UintegralTsProdOutMin=[]  UintegralTsProdOutMax=[]  UngainTsProdOutMin=[]  UngainTsProdOutMax=[]  ClampingZeroOutDataTypeStr=Inherit: Inherit via back propagation  ClampingZeroOutMin=[]  ClampingZeroOutMax=[]  FilterDenConstantOutDataTypeStr=Inherit: Inherit via back propagation  FilterDenConstantOutMin=[]  FilterDenConstantOutMax=[]  PCopyOutDataTypeStr=Inherit: Inherit via back propagation  PCopyOutMin=[]  PCopyOutMax=[]  NCopyOutDataTypeStr=Inherit: Inherit via back propagation  NCopyOutMin=[]  NCopyOutMax=[]  IntegratorContinuousStateAttributes=''  IntegratorStateMustResolveToSignalObject=off  IntegratorRTWStateStorageClass=Auto  FilterContinuousStateAttributes=''  FilterStateMustResolveToSignalObject=off  FilterRTWStateStorageClass=Auto  ParallelPVariant=InternalParameters  IdealPVariant=Disabled  IVariant=InternalParameters  DVariant=InternalParameters  IntegratorVariant=Discrete  SatVariant=Enabled  AWVariant=Passthrough  PCopyVariant=Disabled  TRVariant=Disabled  FdbkBlocksVariant=Forward  IdealPFdbkVariant=Disabled  SatFdbkVariant=Disabled  DerivativeFilterVariant=ForwardEulerFilter  NVariant=InternalParameters  NCopyVariant=Disabled  FilterICVariant=InternalICsFilter  IntegratorICVariant=InternalICs  ExternalResetVariant=Disabled  TRSumVariant=Passthrough  SumFdbkVariant=Disabled  SumVariant=Sum_PID  TsampFilterVariant=InternalTs  TsampNgainVariant=Passthrough  TsampIntegralVariant=Disabled_SignalSpec  ExternalSaturationOutDataTypeStr=Inherit: Same as second input
      settings: LibrarySourceBlock=simulink/Discrete/Discrete PID Controller
  Gain : Gain  Gain=8191  OutDataTypeStr=single
  Multiply : Gain  Gain=TRANS_CH2_7  OutDataTypeStr=single
  Sum : Sum  Inputs=|+-  OutDataTypeStr=single
  Sum1 : Sum  Inputs=|+-  OutDataTypeStr=single
  Sum2 : Sum  Inputs=|++  OutDataTypeStr=single
  Sum3 : Sum  Inputs=|+-  OutDataTypeStr=single
  Sum4 : Sum  Inputs=|++  OutDataTypeStr=single
  Switch1 : Switch  Criteria=u2 > Threshold  Threshold=DEADBAND_CH2_7  OutDataTypeStr=single  SaturateOnIntegerOverflow=off  InputSameDT=off
  Switch2 : Switch  Criteria=u2 > Threshold  Threshold=DEADBAND_CH2_7  OutDataTypeStr=single  SaturateOnIntegerOverflow=off  InputSameDT=off
  Out1 : Outport  OutDataTypeStr=single
  yaw_circle_out : Outport  Port=2  OutDataTypeStr=single
  wires:
  yaw_target/1 -> Sum/1
  Discrete PID Controller1/1 -> Multiply/1
  yaw_circle/1 -> Sum4/2, Gain/1
  Gain/1 -> Sum2/1
  yaw_ecd/1 -> Sum2/2, Sum3/1
  Sum2/1 -> Sum/2
  yaw_last_ecd/1 -> Sum3/2
  Sum3/1 -> Chart1/1(u1)
  Chart1/1(u2) -> Sum4/1
  Sum4/1 -> yaw_circle_out/1
  Multiply/1 -> Sum1/1
  Sum1/1 -> Switch1/1
  yaw_speed_rpm/1 -> Sum1/2
  Discrete PID Controller/1 -> Out1/1
  Switch1/1 -> Discrete PID Controller/1
  Abs/1 -> Switch2/2, Switch1/2
  Constant/1 -> Switch2/3, Switch1/3
  Sum/1 -> Switch2/1, Abs/1
  Switch2/1 -> Discrete PID Controller1/1

== stateflow chart PID_MODEL/Yaw_CH1_5/If Action_speed Subsystem1/Chart1 ==
  state ADD
    en:
    u2 = 1;
    du:
  state IDLE
    en:
    du:
    u2 = 0 ;
  state SUB
    en:
    u2 = -1;
    du:
  (default) -> IDLE
  SUB -> ADD [order 1] : [u1 >= 5000]
  ADD -> IDLE [order 2] : [u1 < 5000 && u1 >-5000]
  ADD -> SUB [order 1] : [u1 <= -5000]
  IDLE -> ADD [order 1] : [u1 >= 5000]
  IDLE -> SUB [order 2] : [u1 <= -5000]
  SUB -> IDLE [order 2] : [u1 < 5000 && u1 >-5000]
  data: u1 input single; u2 output single

== stateflow chart PID_MODEL/Yaw_CH1_6/If Action_speed Subsystem1/Chart1 ==
  state ADD
    en:
    u2 = 1;
    du:
  state IDLE
    en:
    du:
    u2 = 0 ;
  state SUB
    en:
    u2 = -1;
    du:
  (default) -> IDLE
  SUB -> ADD [order 1] : [u1 >= 5000]
  ADD -> IDLE [order 2] : [u1 < 5000 && u1 >-5000]
  ADD -> SUB [order 1] : [u1 <= -5000]
  IDLE -> ADD [order 1] : [u1 >= 5000]
  IDLE -> SUB [order 2] : [u1 <= -5000]
  SUB -> IDLE [order 2] : [u1 < 5000 && u1 >-5000]
  data: u1 input single; u2 output single

== stateflow chart PID_MODEL/Yaw_CH1_7/If Action_speed Subsystem1/Chart1 ==
  state ADD
    en:
    u2 = 1;
    du:
  state IDLE
    en:
    du:
    u2 = 0 ;
  state SUB
    en:
    u2 = -1;
    du:
  (default) -> IDLE
  SUB -> ADD [order 1] : [u1 >= 5000]
  ADD -> IDLE [order 2] : [u1 < 5000 && u1 >-5000]
  ADD -> SUB [order 1] : [u1 <= -5000]
  IDLE -> ADD [order 1] : [u1 >= 5000]
  IDLE -> SUB [order 2] : [u1 <= -5000]
  SUB -> IDLE [order 2] : [u1 < 5000 && u1 >-5000]
  data: u1 input single; u2 output single

== stateflow chart PID_MODEL/Yaw_CH2_2/If Action_speed Subsystem1/Chart1 ==
  state ADD
    en:
    u2 = 1;
    du:
  state IDLE
    en:
    du:
    u2 = 0 ;
  state SUB
    en:
    u2 = -1;
    du:
  (default) -> IDLE
  SUB -> ADD [order 1] : [u1 >= 5000]
  ADD -> IDLE [order 2] : [u1 < 5000 && u1 >-5000]
  ADD -> SUB [order 1] : [u1 <= -5000]
  IDLE -> ADD [order 1] : [u1 >= 5000]
  IDLE -> SUB [order 2] : [u1 <= -5000]
  SUB -> IDLE [order 2] : [u1 < 5000 && u1 >-5000]
  data: u1 input single; u2 output single

== stateflow chart PID_MODEL/Yaw_CH2_3/If Action_speed Subsystem1/Chart1 ==
  state ADD
    en:
    u2 = 1;
    du:
  state IDLE
    en:
    du:
    u2 = 0 ;
  state SUB
    en:
    u2 = -1;
    du:
  (default) -> IDLE
  SUB -> ADD [order 1] : [u1 >= 5000]
  ADD -> IDLE [order 2] : [u1 < 5000 && u1 >-5000]
  ADD -> SUB [order 1] : [u1 <= -5000]
  IDLE -> ADD [order 1] : [u1 >= 5000]
  IDLE -> SUB [order 2] : [u1 <= -5000]
  SUB -> IDLE [order 2] : [u1 < 5000 && u1 >-5000]
  data: u1 input single; u2 output single

== stateflow chart PID_MODEL/Yaw_CH2_4/If Action_speed Subsystem1/Chart1 ==
  state ADD
    en:
    u2 = 1;
    du:
  state IDLE
    en:
    du:
    u2 = 0 ;
  state SUB
    en:
    u2 = -1;
    du:
  (default) -> IDLE
  SUB -> ADD [order 1] : [u1 >= 5000]
  ADD -> IDLE [order 2] : [u1 < 5000 && u1 >-5000]
  ADD -> SUB [order 1] : [u1 <= -5000]
  IDLE -> ADD [order 1] : [u1 >= 5000]
  IDLE -> SUB [order 2] : [u1 <= -5000]
  SUB -> IDLE [order 2] : [u1 < 5000 && u1 >-5000]
  data: u1 input single; u2 output single

== stateflow chart PID_MODEL/Yaw_CH2_5/If Action_speed Subsystem1/Chart1 ==
  state ADD
    en:
    u2 = 1;
    du:
  state IDLE
    en:
    du:
    u2 = 0 ;
  state SUB
    en:
    u2 = -1;
    du:
  (default) -> IDLE
  SUB -> ADD [order 1] : [u1 >= 5000]
  ADD -> IDLE [order 2] : [u1 < 5000 && u1 >-5000]
  ADD -> SUB [order 1] : [u1 <= -5000]
  IDLE -> ADD [order 1] : [u1 >= 5000]
  IDLE -> SUB [order 2] : [u1 <= -5000]
  SUB -> IDLE [order 2] : [u1 < 5000 && u1 >-5000]
  data: u1 input single; u2 output single

== stateflow chart PID_MODEL/Yaw_CH2_6/If Action_speed Subsystem1/Chart1 ==
  state ADD
    en:
    u2 = 1;
    du:
  state IDLE
    en:
    du:
    u2 = 0 ;
  state SUB
    en:
    u2 = -1;
    du:
  (default) -> IDLE
  SUB -> ADD [order 1] : [u1 >= 5000]
  ADD -> IDLE [order 2] : [u1 < 5000 && u1 >-5000]
  ADD -> SUB [order 1] : [u1 <= -5000]
  IDLE -> ADD [order 1] : [u1 >= 5000]
  IDLE -> SUB [order 2] : [u1 <= -5000]
  SUB -> IDLE [order 2] : [u1 < 5000 && u1 >-5000]
  data: u1 input single; u2 output single

== stateflow chart PID_MODEL/Yaw_CH2_7/If Action_speed Subsystem1/Chart1 ==
  state ADD
    en:
    u2 = 1;
    du:
  state IDLE
    en:
    du:
    u2 = 0 ;
  state SUB
    en:
    u2 = -1;
    du:
  (default) -> IDLE
  SUB -> ADD [order 1] : [u1 >= 5000]
  ADD -> IDLE [order 2] : [u1 < 5000 && u1 >-5000]
  ADD -> SUB [order 1] : [u1 <= -5000]
  IDLE -> ADD [order 1] : [u1 >= 5000]
  IDLE -> SUB [order 2] : [u1 <= -5000]
  SUB -> IDLE [order 2] : [u1 < 5000 && u1 >-5000]
  data: u1 input single; u2 output single

== stateflow chart PID_MODEL/Yaw_CH1_1/If Action_speed Subsystem1/Chart1 ==
  state ADD
    en:
    u2 = 1;
    du:
  state IDLE
    en:
    du:
    u2 = 0 ;
  state SUB
    en:
    u2 = -1;
    du:
  (default) -> IDLE
  SUB -> ADD [order 1] : [u1 >= 5000]
  ADD -> IDLE [order 2] : [u1 < 5000 && u1 >-5000]
  ADD -> SUB [order 1] : [u1 <= -5000]
  IDLE -> ADD [order 1] : [u1 >= 5000]
  IDLE -> SUB [order 2] : [u1 <= -5000]
  SUB -> IDLE [order 2] : [u1 < 5000 && u1 >-5000]
  data: u1 input single; u2 output single

== stateflow chart PID_MODEL/Yaw_CH1_2/If Action_speed Subsystem1/Chart1 ==
  state ADD
    en:
    u2 = 1;
    du:
  state IDLE
    en:
    du:
    u2 = 0 ;
  state SUB
    en:
    u2 = -1;
    du:
  (default) -> IDLE
  SUB -> ADD [order 1] : [u1 >= 5000]
  ADD -> IDLE [order 2] : [u1 < 5000 && u1 >-5000]
  ADD -> SUB [order 1] : [u1 <= -5000]
  IDLE -> ADD [order 1] : [u1 >= 5000]
  IDLE -> SUB [order 2] : [u1 <= -5000]
  SUB -> IDLE [order 2] : [u1 < 5000 && u1 >-5000]
  data: u1 input single; u2 output single

== stateflow chart PID_MODEL/Yaw_CH2_1/If Action_speed Subsystem1/Chart1 ==
  state ADD
    en:
    u2 = 1;
    du:
  state IDLE
    en:
    du:
    u2 = 0 ;
  state SUB
    en:
    u2 = -1;
    du:
  (default) -> IDLE
  SUB -> ADD [order 1] : [u1 >= 5000]
  ADD -> IDLE [order 2] : [u1 < 5000 && u1 >-5000]
  ADD -> SUB [order 1] : [u1 <= -5000]
  IDLE -> ADD [order 1] : [u1 >= 5000]
  IDLE -> SUB [order 2] : [u1 <= -5000]
  SUB -> IDLE [order 2] : [u1 < 5000 && u1 >-5000]
  data: u1 input single; u2 output single

== stateflow chart PID_MODEL/Yaw_CH1_3/If Action_speed Subsystem1/Chart1 ==
  state ADD
    en:
    u2 = 1;
    du:
  state IDLE
    en:
    du:
    u2 = 0 ;
  state SUB
    en:
    u2 = -1;
    du:
  (default) -> IDLE
  SUB -> ADD [order 1] : [u1 >= 5000]
  ADD -> IDLE [order 2] : [u1 < 5000 && u1 >-5000]
  ADD -> SUB [order 1] : [u1 <= -5000]
  IDLE -> ADD [order 1] : [u1 >= 5000]
  IDLE -> SUB [order 2] : [u1 <= -5000]
  SUB -> IDLE [order 2] : [u1 < 5000 && u1 >-5000]
  data: u1 input single; u2 output single

== stateflow chart PID_MODEL/Yaw_CH1_4/If Action_speed Subsystem1/Chart1 ==
  state ADD
    en:
    u2 = 1;
    du:
  state IDLE
    en:
    du:
    u2 = 0 ;
  state SUB
    en:
    u2 = -1;
    du:
  (default) -> IDLE
  SUB -> ADD [order 1] : [u1 >= 5000]
  ADD -> IDLE [order 2] : [u1 < 5000 && u1 >-5000]
  ADD -> SUB [order 1] : [u1 <= -5000]
  IDLE -> ADD [order 1] : [u1 >= 5000]
  IDLE -> SUB [order 2] : [u1 <= -5000]
  SUB -> IDLE [order 2] : [u1 < 5000 && u1 >-5000]
  data: u1 input single; u2 output single
